simulink model "simulink1"  (Simulink 7.1)
settings: Solver=ode45  StartTime=0.0  StopTime=10.0  MaxStep=0.1  MinStep=0.001  RelTol=1e-3
settings Model: Creator=surbaniak  LastModifiedBy=surbaniak

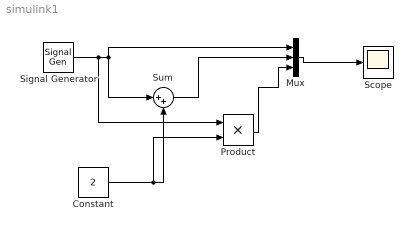
== system simulink1 ==
  Constant : Constant  Value=2  OutDataType=sfix(16)  OutScaling=2^0
  Mux : Mux  Inputs=3
  Product : Product  OutDataType=sfix(16)  OutScaling=2^0  RndMeth=Zero
  Scope : Scope
  Signal Generator : SignalGenerator
  Sum : Sum  Inputs=|++  OutDataType=sfix(16)  OutScaling=2^0
  wires:
  Signal Generator/1 -> Sum/1, Mux/1, Product/1
  Constant/1 -> Sum/2, Product/2
  Sum/1 -> Mux/2
  Mux/1 -> Scope/1
  Product/1 -> Mux/3
